simulink model "IFSSIM_Powertrain"  (R2025b)
settings: Solver=FixedStepDiscrete  StartTime=0  StopTime=inf  FixedStep=1/960  RelTol=1e-3
undefined symbols (not defined in the file): IFSSIM_PowertrainBus_zero
settings Model: Creator=raulmoran  LastModifiedBy=raulmoran

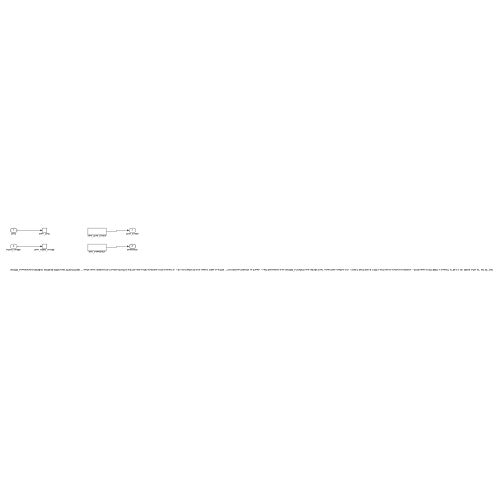
[thumbnail: Simulink's stored preview of the top-level diagram]
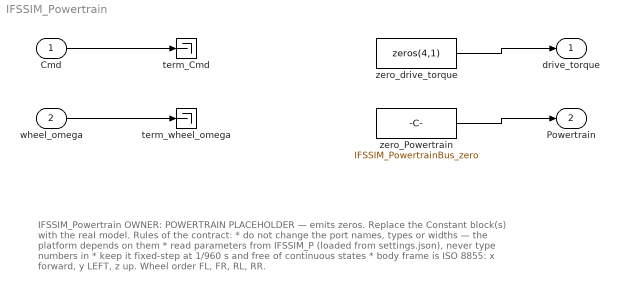
== system IFSSIM_Powertrain ==
  note: IFSSIM_Powertrain\n\nOWNER: POWERTRAIN\n\nPLACEHOLDER — emits zeros. Replace the Constant block(s) with the real model.\n\nRules of the contract:\n * do not change the port names, types or widths — the platform depends on them\n * read parameters from IFSSIM_P (loaded from settings.json), never type numbers in\n * keep it fixed-step at 1/960 s and free of continuous states\n * body frame is ISO 8855: x forward, y LEFT, z up. Wheel order FL, FR, RL, RR.
  Cmd : Inport  OutDataTypeStr=Bus: IFSSIM_CmdBus  BusOutputAsStruct=on
  wheel_omega : Inport  Port=2  PortDimensions=4
  term_Cmd : Terminator
  term_wheel_omega : Terminator
  zero_Powertrain : Constant  Value=IFSSIM_PowertrainBus_zero  OutDataTypeStr=Bus: IFSSIM_PowertrainBus
  zero_drive_torque : Constant  Value=zeros(4,1)
  drive_torque : Outport  PortDimensions=4
  Powertrain : Outport  Port=2  OutDataTypeStr=Bus: IFSSIM_PowertrainBus
  wires:
  Cmd/1 -> term_Cmd/1
  wheel_omega/1 -> term_wheel_omega/1
  zero_drive_torque/1 -> drive_torque/1
  zero_Powertrain/1 -> Powertrain/1
